simulink model "Tf"  (R2023a)
settings: Solver=VariableStepAuto  StartTime=0.0  StopTime=10.0  RelTol=1e-3
settings Model: Creator=13524  LastModifiedBy=13524

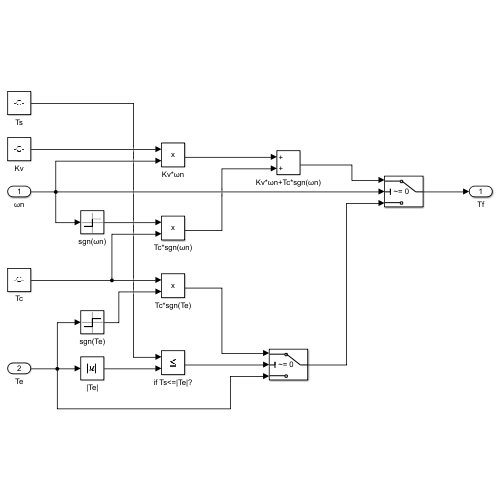
[thumbnail: Simulink's stored preview of the top-level diagram]
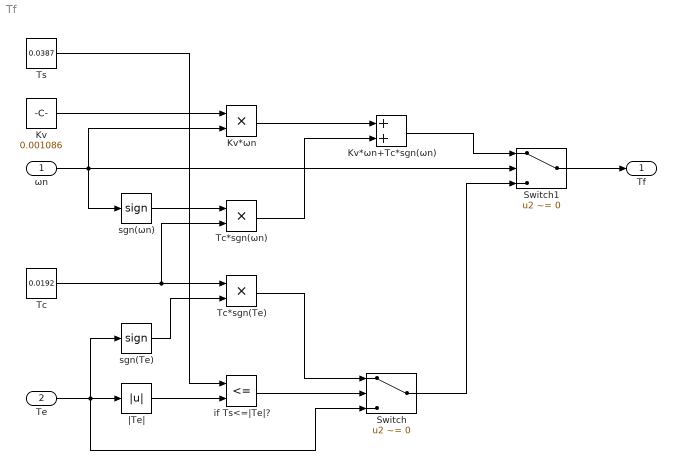
== system Tf ==
  ωn : Inport
  Te : Inport  Port=2
  Kv : Constant  Value=0.001086
  Kv*ωn : Product
  Kv*ωn+Tc*sgn(ωn) : Sum
  Switch : Switch  Criteria=u2 ~= 0  SaturateOnIntegerOverflow=off  InputSameDT=off
  Switch1 : Switch  Criteria=u2 ~= 0  SaturateOnIntegerOverflow=off  InputSameDT=off
  Tc : Constant  Value=0.0192
  Tc*sgn(Te) : Product
  Tc*sgn(ωn) : Product
  Ts : Constant  Value=0.0387
  if Ts<=|Te|? : RelationalOperator  Operator=<=  OutDataTypeStr=boolean  RndMeth=Simplest  InputSameDT=off
  sgn(Te) : Signum
  sgn(ωn) : Signum
  |Te| : Abs  SaturateOnIntegerOverflow=off
  Tf : Outport
  wires:
  Ts/1 -> if Ts<=|Te|?/1
  Te/1 -> Switch/3, sgn(Te)/1, |Te|/1
  |Te|/1 -> if Ts<=|Te|?/2
  if Ts<=|Te|?/1 -> Switch/2
  Tc/1 -> Tc*sgn(ωn)/2, Tc*sgn(Te)/1
  sgn(Te)/1 -> Tc*sgn(Te)/2
  Tc*sgn(Te)/1 -> Switch/1
  ωn/1 -> Switch1/2, sgn(ωn)/1, Kv*ωn/2
  Kv/1 -> Kv*ωn/1
  Kv*ωn/1 -> Kv*ωn+Tc*sgn(ωn)/1
  sgn(ωn)/1 -> Tc*sgn(ωn)/1
  Tc*sgn(ωn)/1 -> Kv*ωn+Tc*sgn(ωn)/2
  Kv*ωn+Tc*sgn(ωn)/1 -> Switch1/1
  Switch/1 -> Switch1/3
  Switch1/1 -> Tf/1
